simulink library "RTC"  (R2022b)
settings: Solver=VariableStepAuto  StartTime=0.0  StopTime=10.0  RelTol=1e-3
undefined symbols (not defined in the file or in its folder): MessagePath, NTF, REQ, RSP, RTC_Mask, unpackedNameList
settings Model: MAModelExclusionFileProxy=C:\work\talariaDev\module\talaria_check_exclusions.xml  Creator=kl13806  LastModifiedBy=kl13806
settings SolverCC: AlgebraicLoopSolver=TrustRegion
settings DebuggingCC: UnconnectedInputMsg=warning  UnconnectedOutputMsg=warning  UnconnectedLineMsg=warning  SFMachineParentedDataDiag=warning  ArithmeticOperatorsInVariantConditions=warning
settings ModelReferenceCC: EnableRefExpFcnMdlSchedulingChecks=on
settings SFSimCC: SimUseLocalCustomCode=off  CustomCodeUndefinedFunction=UseInterfaceOnly
settings RTWCC: TLCOptions=-aINCLUDE_RTC_CONSOLE=1  RTWUseLocalCustomCode=off  DLArmComputeVersion=19.05
settings CodeAppCC: StateflowObjectComments=on

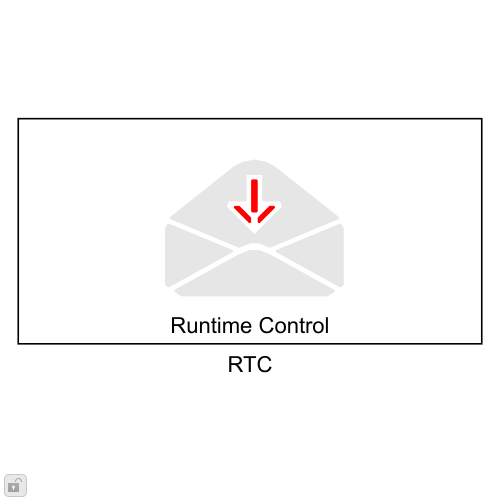
[thumbnail: Simulink's stored preview of the top-level diagram]
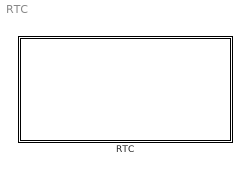
== system RTC ==
  RTC : Subsystem  mask(Talaria RTC Receive){MaskMessageName=, REQ_Priority=RTC_Mask.NormalPriority, RequestAtInit=off, TriggerInit=[-245 -126 -35 -24], EnableRequest=off, REQElemName1=, REQElemType1=uint32, REQElemWidth1=1, REQElemInitial1=[], REQElemName2=, REQElemType2=uint32, REQElemWidth2=1, REQElemInitial2=[], REQElemName3=, REQElemType3=uint32, REQElemWidth3=1, REQElemInitial3=[], REQElemName4=, REQElemType4=uint32, REQElemWidth4=1, REQElemInitial4=[], REQElemName5=, REQElemType5=uint32, REQElemWidth5=1, REQElemInitial5=[], REQElemName6=, REQElemType6=uint32, REQElemWidth6=1, REQElemInitial6=[], REQElemName7=, REQElemType7=uint32, REQElemWidth7=1, REQElemInitial7=[], REQElemName8=, REQElemType8=uint32, REQElemWidth8=1, REQElemInitial8=[], REQElemName9=, REQElemType9=uint32, REQElemWidth9=1, REQElemInitial9=[], REQElemName10=, REQElemType10=uint32, REQElemWidth10=1, REQElemInitial10=[], EnableResponse=off, EnableRSP_StatusIn=off, RSPElemName1=, RSPElemType1=uint32, RSPElemWidth1=1, RSPElemName2=, RSPElemType2=uint32, RSPElemWidth2=1, RSPElemName3=, RSPElemType3=uint32, RSPElemWidth3=1, RSPElemName4=, RSPElemType4=uint32, RSPElemWidth4=1, RSPElemName5=, RSPElemType5=uint32, RSPElemWidth5=1, RSPElemName6=, RSPElemType6=uint32, RSPElemWidth6=1, RSPElemName7=, RSPElemType7=uint32, RSPElemWidth7=1, RSPElemName8=, RSPElemType8=uint32, RSPElemWidth8=1, RSPElemName9=, RSPElemType9=uint32, RSPElemWidth9=1, RSPElemName10=, RSPElemType10=uint32, RSPElemWidth10=1, EnableNotification=off, EnableNTF_PrepTrig=off, NTFElemName1=, NTFElemType1=uint32, NTFElemWidth1=1, NTFElemName2=, NTFElemType2=uint32, NTFElemWidth2=1, NTFElemName3=, NTFElemType3=uint32, NTFElemWidth3=1, NTFElemName4=, NTFElemType4=uint32, NTFElemWidth4=1, NTFElemName5=, NTFElemType5=uint32, NTFElemWidth5=1, NTFElemName6=, NTFElemType6=uint32, NTFElemWidth6=1, NTFElemName7=, NTFElemType7=uint32, NTFElemWidth7=1, NTFElemName8=, NTFElemType8=uint32, NTFElemWidth8=1, NTFElemName9=, NTFElemType9=uint32, NTFElemWidth9=1, NTFElemName10=, NTFElemType10=uint32, NTFElemWidth10=1}
      mask prompts: MaskMessageName "Message name"; REQ_Priority "Priority (0=normal, 1=high)"; RequestAtInit "Trigger request handler during initialization."; TriggerInit "(non-visible trigger param)"; EnableRequest "Output Request/Response function trigger"; EnableResponse "Generate Response Payload"; EnableRSP_StatusIn "Input a status code"; EnableNotification "(Reponse payload must be enabled to allow notifications)"; EnableNTF_PrepTrig "Output NTF prep trigger"
      mask help: This block receives control messages at runtime that inject dynamic configuration settings into the model. Typically the control messages originate from an external source such as a volume knob, a vehicle network signal, or a microcontroller diagnostic control.
      mask init:
      | % Bit-masks for debug printfs. (e.g. bit 0x8 is to debug simulation)
      | DbgTriggerREQRSP = hex2dec('0');
      | DbgTriggerNTF    = hex2dec('0');
      | DebugBytePackREQ = hex2dec('0');
      | DebugBytePackRSP = hex2dec('0');
      | DebugBytePackNTF = hex2dec('0');
      | rtcH = gcbh;
      | 
      | % Register and pull out the parts of our various payloads
      | [ok,okToWire,MessagePath,REQ,RSP,NTF,indirectAddressing,payloadMetaHash] = ...
      |    RTC_Mask.InitPayloadDefinitions(rtcH);
      | 
      | if (okToWire)
      |    RTC_Mask.InitWireSystem(rtcH,MessagePath,REQ,RSP,NTF);
      | end
      | 
      | coreIndex = CoreIndexMask.GetCoreIndex(rtcH);
      | 
      | % Share our description with sub blocks (RTC REQ RSP trigger)
      | Description = get_param(rtcH,'Description');
      settings: MoveFcn=RTC_Mask.CB_TriggerInit(gcbh);
      mask Help:
      | The RTC Receive block provides Run Time Control of algorithms similar to the "UserControlCode" mechanism present in hand written systems. RTC services offer a protocol of communication that includes a request, a response, and an optional notification. The RTC block mask parameters specify the content of the payload for each of these types of message. Open the mask parameters to add elements to the various payload types and specify whether or not a notification payload is generated for this block.
      | 
      | <u>Message Payloads:</u>
      | The Request, or "<b>REQ</b>" : the request message originates from control logic (e.g. a microcontroller). Add elements to the request payload similar to the arguments of a function call. For example, a target gain level and a ramp time would make appropriate REQ signals to request a volume change. The RTC block provides a function trigger output signal useful to trigger any logic required to interpret the request payload and kick off actions.
      | 
      | The Response, or "<b>RSP</b>" : the response message returns at once from the algorithm to confirm receipt of the request. The You may add signals to the response message payload as well if there are properties immediately available at the time of the request. The same function trigger used to receive the request can be used to calculate or acquire signals for the response payload. Perhaps the RTC block's "REQ_trigger" output should really be named the "REQ_RSP_trigger". For example, a current gain level would make an appropriate RSP signal to a request to get the current gain level.
      | If a response is defined for a block, then its request payload automatically includes a caller handle used to match responses (and notifications) to their original request. The caller handle is not used by the algorithmic logic, so it never appears as a signal coming out of the RTC block. However, simulated request payloads (see below) must also include a caller handle.
      | 
      | The Notification,  or "<b>NTF</b>" : the notification message is optionally enabled for each RTC service. When enabled, the algorithm is able to send a follow up response to a request some time later. For example, a notification message could be sent once a gain change request has finally reached the target gain after several milliseconds. Note that even when notifications are enabled for an RTC service, not *every* request is gauranteed to receive a notification. Consider a fast series of the same request received in succession by the algorithm.  The earlier requests may be prevented from completing their task and emitting a notification because subsequent requests have changed the target. Depending on an algorithm's implementation, only requests that are allowed to finish their task uninterrupted will be able to emit a notification.
      | 
      | <u>Simulated Requests and Simulation:</u>
      | The RTC_SimData class collaborates with RTC blocks during simulation to simlate transfer of RTC message payloads. RTC blocks look for a global instance of RTC_SimData called "RTC_SIM_OBJ" during simulation. The IntFcn callback at the model level is a recommended place to load simulated RTC messages (e.g. via invocation of a script). Here's an example script that sets up two simulated RTC events:
      | 	RTC_SIM_OBJ = RTC_SimData(10);			% pre-allocate for 10 messages
      | 	RTC_SIM_OBJ.AddREQ( 'Preamp_SetVolume', 0.5, [451 255, 1000 0]);	% at simulation time 0.5, make a request (with a caller handle of '451') to set the volume to index 255 with ramp arguments of 1000 and 0.
      | 	RTC_SIM_OBJ.AddREQ( 'Preamp_SetMute', 2, [23 1]);	% mute everything 2 seconds into the simulation (caller handle is '23')
      | 
      | Simulated RTC payloads are fed from a simple single array of numeric values as shown above. Any RTC payload elements with a width greater than one will just claim more values from the array. In other words, if an RTC message has a payload with scalar first element and a second vector element of width 2, the simulated payload should be an array of length 3.
      | 
      | After simulation completes, open up the RTC_SimData object (i.e. 'open RTC_SIM_OBJ') to investigate the simulated response and notification messages.
      | 
      | <u>Advanced Settings</u>
      | <b>Priority</b> supports either high or low priority as represented by a bit embedded into the message token generated for each RTC service. The intent is that during platform integration, high priority RTC requests could be handled by a higher priority thread. This capability relies on support from platform integration. Please note that high priority requests should *not* attempt to return a notification due to race conditions since there is no high-priority notification service. High priority RTC messages are best for streaming periodic signals like vehicle engine speed - low latency simple data with no significant processing upon receipt.
      | 
      | <b>Trigger request handler during initialization</b> when selected will execute the RTC request trigger whenever the RTC block is enabled. This happens at startup or anytime the containing subsystem is enabled if part of an enabled subsystem. The request payload values that are used during this enable execution are power-on defaults or the last-received request from control code. Please note a high likelihood of hard-to-detect failure if the logic triggered by the RTC request includes blocks which themselves include data initialization. For instance, a MATLAB function block with persistent data that is triggered by request will likely initialize the persistent data AFTER the RTC handler is called at initialization. Behavior is different here between code generation and model simulation. Similarly, if any signals fed to the triggered logic are "live" signals that change or buffers that support reuse, then the data present during initiation handling will be unreliable. TOP inputs are safe for code generation. Using TOP inputs in a "source model" will only receive valid TOPs on the SECOND simulation since TuneVar->TOP translations are run after initialization during the start of simulation.
      mask Callback TriggerInit: RTC_Mask.CB_TriggerInit(gcbh);
      mask Callback EnableRequest: RTC_Mask.CB_EnableRequest(gcbh);
      mask Callback REQElemName1: RTC_Mask.CB_ElemName(gcbh,'REQ','1');
      mask TypeOptions REQElemType1: double | single | int8 | uint8 | int16 | uint16 | int32 | uint32 | boolean
      mask Callback REQElemWidth1: RTC_Mask.CB_ElemWidth(gcbh,'REQ','1');
      mask Callback REQElemInitial1: RTC_Mask.CB_ElemInitial(gcbh,'REQ','1');
      mask Callback REQElemName2: RTC_Mask.CB_ElemName(gcbh,'REQ','2');
      mask TypeOptions REQElemType2: double | single | int8 | uint8 | int16 | uint16 | int32 | uint32 | boolean
      mask Callback REQElemWidth2: RTC_Mask.CB_ElemWidth(gcbh,'REQ','2');
      mask Callback REQElemInitial2: RTC_Mask.CB_ElemInitial(gcbh,'REQ','2');
      mask Callback REQElemName3: RTC_Mask.CB_ElemName(gcbh,'REQ','3');
      mask TypeOptions REQElemType3: double | single | int8 | uint8 | int16 | uint16 | int32 | uint32 | boolean
      mask Callback REQElemWidth3: RTC_Mask.CB_ElemWidth(gcbh,'REQ','3');
      mask Callback REQElemInitial3: RTC_Mask.CB_ElemInitial(gcbh,'REQ','3');
      mask Callback REQElemName4: RTC_Mask.CB_ElemName(gcbh,'REQ','4');
      mask TypeOptions REQElemType4: double | single | int8 | uint8 | int16 | uint16 | int32 | uint32 | boolean
      mask Callback REQElemWidth4: RTC_Mask.CB_ElemWidth(gcbh,'REQ','4');
      mask Callback REQElemInitial4: RTC_Mask.CB_ElemInitial(gcbh,'REQ','4');
      mask Callback REQElemName5: RTC_Mask.CB_ElemName(gcbh,'REQ','5');
      mask TypeOptions REQElemType5: double | single | int8 | uint8 | int16 | uint16 | int32 | uint32 | boolean
      mask Callback REQElemWidth5: RTC_Mask.CB_ElemWidth(gcbh,'REQ','5');
      mask Callback REQElemInitial5: RTC_Mask.CB_ElemInitial(gcbh,'REQ','5');
      mask Callback REQElemName6: RTC_Mask.CB_ElemName(gcbh,'REQ','6');
      mask TypeOptions REQElemType6: double | single | int8 | uint8 | int16 | uint16 | int32 | uint32 | boolean
      mask Callback REQElemWidth6: RTC_Mask.CB_ElemWidth(gcbh,'REQ','6');
      mask Callback REQElemInitial6: RTC_Mask.CB_ElemInitial(gcbh,'REQ','6');
      mask Callback REQElemName7: RTC_Mask.CB_ElemName(gcbh,'REQ','7');
      mask TypeOptions REQElemType7: double | single | int8 | uint8 | int16 | uint16 | int32 | uint32 | boolean
      mask Callback REQElemWidth7: RTC_Mask.CB_ElemWidth(gcbh,'REQ','7');
      mask Callback REQElemInitial7: RTC_Mask.CB_ElemInitial(gcbh,'REQ','7');
      mask Callback REQElemName8: RTC_Mask.CB_ElemName(gcbh,'REQ','8');
      mask TypeOptions REQElemType8: double | single | int8 | uint8 | int16 | uint16 | int32 | uint32 | boolean
      mask Callback REQElemWidth8: RTC_Mask.CB_ElemWidth(gcbh,'REQ','8');
      mask Callback REQElemInitial8: RTC_Mask.CB_ElemInitial(gcbh,'REQ','8');
      mask Callback REQElemName9: RTC_Mask.CB_ElemName(gcbh,'REQ','9');
      mask TypeOptions REQElemType9: double | single | int8 | uint8 | int16 | uint16 | int32 | uint32 | boolean
      mask Callback REQElemWidth9: RTC_Mask.CB_ElemWidth(gcbh,'REQ','9');
      mask Callback REQElemInitial9: RTC_Mask.CB_ElemInitial(gcbh,'REQ','9');
      mask Callback REQElemName10: RTC_Mask.CB_ElemName(gcbh,'REQ','10');
      mask TypeOptions REQElemType10: double | single | int8 | uint8 | int16 | uint16 | int32 | uint32 | boolean
      mask Callback REQElemWidth10: RTC_Mask.CB_ElemWidth(gcbh,'REQ','10');
      mask Callback REQElemInitial10: RTC_Mask.CB_ElemInitial(gcbh,'REQ','10');
      mask Callback EnableResponse: RTC_Mask.CB_EnableResponse(gcbh);
      mask Callback EnableRSP_StatusIn: RTC_Mask.CB_EnableRSP_StatusIn(gcbh);
      mask Callback RSPElemName1: RTC_Mask.CB_ElemName(gcbh,'RSP','1');
      mask TypeOptions RSPElemType1: double | single | int8 | uint8 | int16 | uint16 | int32 | uint32 | boolean
      mask Callback RSPElemWidth1: RTC_Mask.CB_ElemWidth(gcbh,'RSP','1');
      mask Callback RSPElemName2: RTC_Mask.CB_ElemName(gcbh,'RSP','2');
      mask TypeOptions RSPElemType2: double | single | int8 | uint8 | int16 | uint16 | int32 | uint32 | boolean
      mask Callback RSPElemWidth2: RTC_Mask.CB_ElemWidth(gcbh,'RSP','2');
      mask Callback RSPElemName3: RTC_Mask.CB_ElemName(gcbh,'RSP','3');
      mask TypeOptions RSPElemType3: double | single | int8 | uint8 | int16 | uint16 | int32 | uint32 | boolean
      mask Callback RSPElemWidth3: RTC_Mask.CB_ElemWidth(gcbh,'RSP','3');
      mask Callback RSPElemName4: RTC_Mask.CB_ElemName(gcbh,'RSP','4');
      mask TypeOptions RSPElemType4: double | single | int8 | uint8 | int16 | uint16 | int32 | uint32 | boolean
      mask Callback RSPElemWidth4: RTC_Mask.CB_ElemWidth(gcbh,'RSP','4');
      mask Callback RSPElemName5: RTC_Mask.CB_ElemName(gcbh,'RSP','5');
      mask TypeOptions RSPElemType5: double | single | int8 | uint8 | int16 | uint16 | int32 | uint32 | boolean
      mask Callback RSPElemWidth5: RTC_Mask.CB_ElemWidth(gcbh,'RSP','5');
      mask Callback RSPElemName6: RTC_Mask.CB_ElemName(gcbh,'RSP','6');
      mask TypeOptions RSPElemType6: double | single | int8 | uint8 | int16 | uint16 | int32 | uint32 | boolean
      mask Callback RSPElemWidth6: RTC_Mask.CB_ElemWidth(gcbh,'RSP','6');
      mask Callback RSPElemName7: RTC_Mask.CB_ElemName(gcbh,'RSP','7');
      mask TypeOptions RSPElemType7: double | single | int8 | uint8 | int16 | uint16 | int32 | uint32 | boolean
      mask Callback RSPElemWidth7: RTC_Mask.CB_ElemWidth(gcbh,'RSP','7');
      mask Callback RSPElemName8: RTC_Mask.CB_ElemName(gcbh,'RSP','8');
      mask TypeOptions RSPElemType8: double | single | int8 | uint8 | int16 | uint16 | int32 | uint32 | boolean
      mask Callback RSPElemWidth8: RTC_Mask.CB_ElemWidth(gcbh,'RSP','8');
      mask Callback RSPElemName9: RTC_Mask.CB_ElemName(gcbh,'RSP','9');
      mask TypeOptions RSPElemType9: double | single | int8 | uint8 | int16 | uint16 | int32 | uint32 | boolean
      mask Callback RSPElemWidth9: RTC_Mask.CB_ElemWidth(gcbh,'RSP','9');
      mask Callback RSPElemName10: RTC_Mask.CB_ElemName(gcbh,'RSP','10');
      mask TypeOptions RSPElemType10: double | single | int8 | uint8 | int16 | uint16 | int32 | uint32 | boolean
      mask Callback RSPElemWidth10: RTC_Mask.CB_ElemWidth(gcbh,'RSP','10');
      mask Callback EnableNotification: RTC_Mask.CB_EnableNotification(gcbh);
      mask Callback EnableNTF_PrepTrig: RTC_Mask.CB_EnableNTF_PrepTrig(gcbh);
      mask Callback NTFElemName1: RTC_Mask.CB_ElemName(gcbh,'NTF','1');
      mask TypeOptions NTFElemType1: double | single | int8 | uint8 | int16 | uint16 | int32 | uint32 | boolean
      mask Callback NTFElemWidth1: RTC_Mask.CB_ElemWidth(gcbh,'NTF','1');
      mask Callback NTFElemName2: RTC_Mask.CB_ElemName(gcbh,'NTF','2');
      mask TypeOptions NTFElemType2: double | single | int8 | uint8 | int16 | uint16 | int32 | uint32 | boolean
      mask Callback NTFElemWidth2: RTC_Mask.CB_ElemWidth(gcbh,'NTF','2');
      mask Callback NTFElemName3: RTC_Mask.CB_ElemName(gcbh,'NTF','3');
      mask TypeOptions NTFElemType3: double | single | int8 | uint8 | int16 | uint16 | int32 | uint32 | boolean
      mask Callback NTFElemWidth3: RTC_Mask.CB_ElemWidth(gcbh,'NTF','3');
      mask Callback NTFElemName4: RTC_Mask.CB_ElemName(gcbh,'NTF','4');
      mask TypeOptions NTFElemType4: double | single | int8 | uint8 | int16 | uint16 | int32 | uint32 | boolean
      mask Callback NTFElemWidth4: RTC_Mask.CB_ElemWidth(gcbh,'NTF','4');
      mask Callback NTFElemName5: RTC_Mask.CB_ElemName(gcbh,'NTF','5');
      mask TypeOptions NTFElemType5: double | single | int8 | uint8 | int16 | uint16 | int32 | uint32 | boolean
      mask Callback NTFElemWidth5: RTC_Mask.CB_ElemWidth(gcbh,'NTF','5');
      mask Callback NTFElemName6: RTC_Mask.CB_ElemName(gcbh,'NTF','6');
      mask TypeOptions NTFElemType6: double | single | int8 | uint8 | int16 | uint16 | int32 | uint32 | boolean
      mask Callback NTFElemWidth6: RTC_Mask.CB_ElemWidth(gcbh,'NTF','6');
      mask Callback NTFElemName7: RTC_Mask.CB_ElemName(gcbh,'NTF','7');
      mask TypeOptions NTFElemType7: double | single | int8 | uint8 | int16 | uint16 | int32 | uint32 | boolean
      mask Callback NTFElemWidth7: RTC_Mask.CB_ElemWidth(gcbh,'NTF','7');
      mask Callback NTFElemName8: RTC_Mask.CB_ElemName(gcbh,'NTF','8');
      mask TypeOptions NTFElemType8: double | single | int8 | uint8 | int16 | uint16 | int32 | uint32 | boolean
      mask Callback NTFElemWidth8: RTC_Mask.CB_ElemWidth(gcbh,'NTF','8');
      mask Callback NTFElemName9: RTC_Mask.CB_ElemName(gcbh,'NTF','9');
      mask TypeOptions NTFElemType9: double | single | int8 | uint8 | int16 | uint16 | int32 | uint32 | boolean
      mask Callback NTFElemWidth9: RTC_Mask.CB_ElemWidth(gcbh,'NTF','9');
      mask Callback NTFElemName10: RTC_Mask.CB_ElemName(gcbh,'NTF','10');
      mask TypeOptions NTFElemType10: double | single | int8 | uint8 | int16 | uint16 | int32 | uint32 | boolean
      mask Callback NTFElemWidth10: RTC_Mask.CB_ElemWidth(gcbh,'NTF','10');
      mask DialogControl DescriptionPanel Prompt: Description
      mask DialogControl EditDescription Prompt: Edit Description
      mask DialogControl EditDescription Callback: RTC_Mask.CB_EditDescription(gcbh);
      mask DialogControl AdvancedPanel Prompt: Advanced Settings
      mask DialogControl TextInitWarn Prompt: <font color="red">Warning: triggered handler must not include data or process live signals</font>
      mask DialogControl REQTab Prompt: Request Payload
      mask DialogControl REQShowWidth Prompt: Width
      mask DialogControl REQShowWidth Callback: RTC_Mask.CB_ShowInitial(gcbh,'REQ',false);
      mask DialogControl REQShowInitial Prompt: Initial Val
      mask DialogControl REQShowInitial Callback: RTC_Mask.CB_ShowInitial(gcbh,'REQ',true);
      mask DialogControl REQtxtName Prompt: Element name
      mask DialogControl REQtxtType Prompt: Type
      mask DialogControl REQtxtLastCol Prompt: Width
      mask DialogControl REQAddSignal Prompt: Add Signal
      mask DialogControl REQAddSignal Callback: RTC_Mask.CB_AddSignal(gcbh,'REQ');
      mask DialogControl RSPTab Prompt: Response Payload
      mask DialogControl RSPtxtName Prompt: Element name
      mask DialogControl RSPtxtType Prompt: Type
      mask DialogControl RSPtxtLastCol Prompt: Width
      mask DialogControl RSPAddSignal Prompt: Add Signal
      mask DialogControl RSPAddSignal Callback: RTC_Mask.CB_AddSignal(gcbh,'RSP');
      mask DialogControl NTFTab Prompt: Notification Payload
      mask DialogControl NTFtxtName Prompt: Element name
      mask DialogControl NTFtxtType Prompt: Type
      mask DialogControl NTFtxtLastCol Prompt: Width
      mask DialogControl NTFAddSignal Prompt: Add Signal
      mask DialogControl NTFAddSignal Callback: RTC_Mask.CB_AddSignal(gcbh,'NTF');
      mask DialogControl ErrorContainer Prompt: Error Messages
      mask Display:
      | % load icon definition
      | [path,w,h] = RTC_Mask.Icon(REQ_Priority);
      | 
      | % retrieve the block's pixel size
      | pos = get(gcbh,'position');
      | bw = pos(3) - pos(1);
      | bh = pos(4) - pos(2);
      | 
      | % draw centered icon
      | xAdj = bw/2 - w/2;
      | yAdj = bh/2 - h/2 + 6;
      | for i=1:length(path)
      |     patch(path(i).x+xAdj, path(i).y+yAdj, path(i).rgb);
      | end
      | 
      | % show the message path or a big red X when disabled
      | if (exist('ok','var') && ok)
      |         % Display the received message path
      |         text(bw/2, bh*0.02,MessagePath, ...
      |             'horizontalAlignment','center', ...
      |             'VerticalAlignment','bottom');
      |         patch(0,0,[1 1 1]);
      |         patch(bw,bh,[1 1 1]);
      |     else
      |         tx=bw*0.03;
      |         ty=bh*0.03;
      |         patch([0 tx bw bw-tx], [ty 0 bh-ty bh], [1 0 0]);
      |         patch([0 bw-tx bw tx], [bh-ty 0 ty bh], [1 0 0]);
      | end

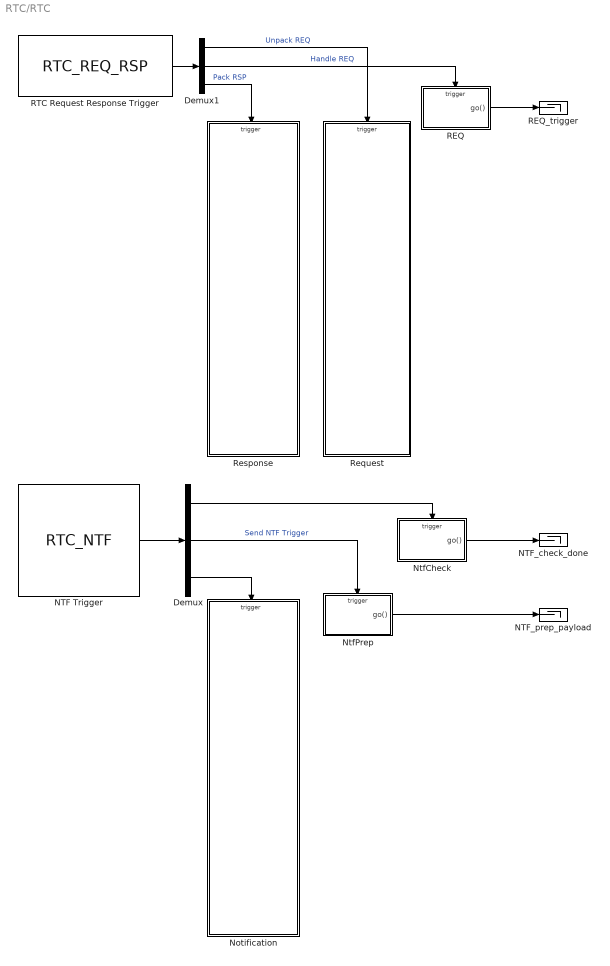
== system RTC/RTC ==
  Demux : Demux  Outputs=3
  Demux1 : Demux  Outputs=3
  NTF Trigger : S-Function  FunctionName=RTC_NTF  Parameters=MessagePath,EnableNotification, NTF.TotalCharSize, DbgTriggerNTF  SFunctionDeploymentMode=off  EnableBusSupport=off
  NTF_check_done : Terminator
  NTF_prep_payload : Terminator
  Notification : Subsystem  TreatAsAtomicUnit=on
  NtfCheck : MATLAB Function  TreatAsAtomicUnit=on
      settings: RTWSystemCode=Inline
  NtfPrep : MATLAB Function  TreatAsAtomicUnit=on
      settings: RTWSystemCode=Inline
  REQ : MATLAB Function  TreatAsAtomicUnit=on  RTWFcnName=RTC_DONOTHING_BLOCK
      settings: RTWSystemCode=Nonreusable function
  REQ_trigger : Terminator
  RTC Request Response Trigger : S-Function  FunctionName=RTC_REQ_RSP  Parameters=MessagePath, coreIndex, REQ_Priority, REQ.TotalCharSize, RSP.TotalCharSize, NTF.TotalCharSize, Description, RequestAtInit, payloadMetaHash, DbgTriggerREQRSP  SFunctionDeploymentMode=off  EnableBusSupport=off
  Request : Subsystem
  Response : Subsystem  TreatAsAtomicUnit=on
  wires:
  Demux/1 -> NtfCheck/Trigger
  Demux/2 -> NtfPrep/Trigger  "Send NTF Trigger"
  Demux/3 -> Notification/Trigger
  RTC Request Response Trigger/1 -> Demux1/1
  NTF Trigger/1 -> Demux/1
  REQ/1(go()) -> REQ_trigger/1
  Demux1/2 -> REQ/Trigger  "Handle REQ"
  Demux1/1 -> Request/Trigger  "Unpack REQ"
  Demux1/3 -> Response/Trigger  "Pack RSP"
  NtfPrep/1(go()) -> NTF_prep_payload/1
  NtfCheck/1(go()) -> NTF_check_done/1

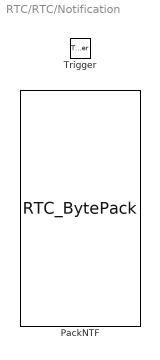
== system RTC/RTC/Notification ==
  Trigger : TriggerPort  TriggerType=function-call  VariantControl=Variant
  PackNTF : S-Function  FunctionName=RTC_BytePack  Parameters=PackedDataName,unpackedNameList,UnpackedTypes,UnpackedWidths,ElemCharIndex,ElemCharSize,TotalCharSize,BlockRole,MessagePath,DebugLevel  SFunctionDeploymentMode=off  EnableBusSupport=off  mask{PackedDataName='pNTFBuf', UnpackedNames=NTF.Name, UnpackedTypes=NTF.TypeId, UnpackedWidths=NTF.Width, ElemCharIndex=NTF.CharIndex, ElemCharSize=NTF.CharSize, TotalCharSize=NTF.TotalCharSize, BlockRole=2, MessagePath=MessagePath, DebugLevel=DebugBytePackNTF}
      mask prompts: PackedDataName "Code variable name for buffer (string)"; UnpackedNames "Unpacked signal names"; UnpackedTypes "Unpacked signal type ids"; UnpackedWidths "Unpacked signal widths"; ElemCharIndex "Starting char index for each signal in packed form"; ElemCharSize "Char size for each signal in packed form"; TotalCharSize "Total char size of packed form including MsgId"; BlockRole "Block role id (0=REQ, 1=RSP, 2=NTF)"; MessagePath "Message feature path"; DebugLevel "Debug level"
      mask help: This block marshals signals either to or from a packed buffer.
      mask init:
      | [unpackedNameList,unpackedStruct] = RTC_BytePackMask.DoInit(PackedDataName,UnpackedNames,UnpackedTypes, ...
      |     UnpackedWidths,ElemCharIndex,ElemCharSize,TotalCharSize,BlockRole, ...
      |     MessagePath,DebugLevel);

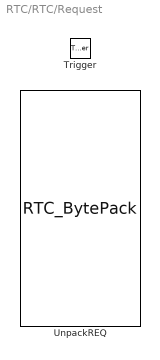
== system RTC/RTC/Request ==
  Trigger : TriggerPort  TriggerType=function-call  VariantControl=Variant
  UnpackREQ : S-Function  FunctionName=RTC_BytePack  Parameters=PackedDataName,unpackedNameList,UnpackedTypes,UnpackedWidths,ElemCharIndex,ElemCharSize,TotalCharSize,BlockRole,MessagePath,DebugLevel  SFunctionDeploymentMode=off  EnableBusSupport=off  mask{PackedDataName='pREQBuf', UnpackedNames=REQ.Name, UnpackedTypes=REQ.TypeId, UnpackedWidths=REQ.Width, ElemCharIndex=REQ.CharIndex, ElemCharSize=REQ.CharSize, TotalCharSize=REQ.TotalCharSize, BlockRole=0, MessagePath=MessagePath, DebugLevel=DebugBytePackREQ}
      mask prompts: PackedDataName "Code variable name for buffer (string)"; UnpackedNames "Unpacked signal names"; UnpackedTypes "Unpacked signal type ids"; UnpackedWidths "Unpacked signal widths"; ElemCharIndex "Starting char index for each signal in packed form"; ElemCharSize "Char size for each signal in packed form"; TotalCharSize "Total char size of packed form including MsgId"; BlockRole "Block role id (0=REQ, 1=RSP, 2=NTF)"; MessagePath "Message feature path"; DebugLevel "Debug level"
      mask help: This block marshals signals either to or from a packed buffer.
      mask init: same as RTC/RTC/Notification/PackNTF

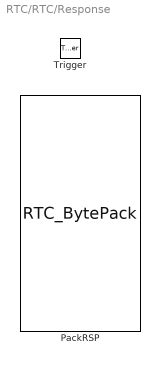
== system RTC/RTC/Response ==
  Trigger : TriggerPort  TriggerType=function-call  VariantControl=Variant
  PackRSP : S-Function  FunctionName=RTC_BytePack  Parameters=PackedDataName,unpackedNameList,UnpackedTypes,UnpackedWidths,ElemCharIndex,ElemCharSize,TotalCharSize,BlockRole,MessagePath,DebugLevel  SFunctionDeploymentMode=off  EnableBusSupport=off  mask{PackedDataName='pRSPBuf', UnpackedNames=RSP.Name, UnpackedTypes=RSP.TypeId, UnpackedWidths=RSP.Width, ElemCharIndex=RSP.CharIndex, ElemCharSize=RSP.CharSize, TotalCharSize=RSP.TotalCharSize, BlockRole=1, MessagePath=MessagePath, DebugLevel=DebugBytePackRSP}
      mask prompts: PackedDataName "Code variable name for buffer (string)"; UnpackedNames "Unpacked signal names"; UnpackedTypes "Unpacked signal type ids"; UnpackedWidths "Unpacked signal widths"; ElemCharIndex "Starting char index for each signal in packed form"; ElemCharSize "Char size for each signal in packed form"; TotalCharSize "Total char size of packed form including MsgId"; BlockRole "Block role id (0=REQ, 1=RSP, 2=NTF)"; MessagePath "Message feature path"; DebugLevel "Debug level"
      mask help: This block marshals signals either to or from a packed buffer.
      mask init: same as RTC/RTC/Notification/PackNTF

== matlab function RTC/REQ ==
  events: go output FUNCTION_CALL_EVENT; trigger input FUNCTION_CALL_EVENT
function func()
% Invoke the function trigger output
go();

== matlab function RTC/NtfPrep ==
  events: go output FUNCTION_CALL_EVENT; trigger input FUNCTION_CALL_EVENT
function func()
% Invoke the function trigger output
go();

== matlab function RTC/NtfCheck ==
  events: go output FUNCTION_CALL_EVENT; trigger input FUNCTION_CALL_EVENT
function func()
% Invoke the function trigger output
go();
